simulink model "FSAC2021_V1"  (R2014a)
settings: Solver=FixedStepDiscrete  StartTime=0.0  StopTime=inf  FixedStep=0.0005  RelTol=1e-3
model workspace (MAT data in the model file):
  MCOS : class17 (value not decoded)
  MCOS : class17 (value not decoded)
  MCOS : class17 (value not decoded)
  MCOS : class17 (value not decoded)
  MCOS : class17 (value not decoded)
  MCOS : class17 (value not decoded)
  MCOS : class17 (value not decoded)
  MCOS : class17 (value not decoded)
  MCOS : class17 (value not decoded)
  MCOS : class17 (value not decoded)
  MCOS : class17 (value not decoded)
  MCOS : class17 (value not decoded)
  MCOS : class17 (value not decoded)
  MCOS : class17 (value not decoded)
  MCOS : class17 (value not decoded)
  MCOS : class17 (value not decoded)
  MCOS : class17 (value not decoded)
  MCOS : class17 (value not decoded)
  MCOS : class17 (value not decoded)
  BUZZER_START = 1
  MCOS : class17 (value not decoded)
  MCOS : class17 (value not decoded)
  MCOS : class17 (value not decoded)
  MCOS : class17 (value not decoded)
  MCOS : class17 (value not decoded)
  MCOS : class17 (value not decoded)
  MCOS : class17 (value not decoded)
  MCOS : class17 (value not decoded)
  MCOS : class17 (value not decoded)
  MCOS : class17 (value not decoded)
  MCOS : class17 (value not decoded)
  MCOS : class17 (value not decoded)
  MCOS : class17 (value not decoded)
  MCOS : class17 (value not decoded)
  MCOS : class17 (value not decoded)
  MCOS : class17 (value not decoded)
  MCOS : class17 (value not decoded)
  MCOS : class17 (value not decoded)
  MCOS : class17 (value not decoded)
  MCOS : class17 (value not decoded)
  MCOS : class17 (value not decoded)
  MCOS : class17 (value not decoded)
  MCOS : class17 (value not decoded)
  MCOS : class17 (value not decoded)
  MCOS : class17 (value not decoded)
  MCOS : class17 (value not decoded)
  MCOS : class17 (value not decoded)
  MCOS : class17 (value not decoded)
  MCOS : class17 (value not decoded)
  MCOS : class17 (value not decoded)
  MCOS : class17 (value not decoded)
  MCOS : class17 (value not decoded)
  MCOS : class17 (value not decoded)
  MCOS : class17 (value not decoded)
  MCOS : class17 (value not decoded)
  MCOS : class17 (value not decoded)
  MCOS : class17 (value not decoded)
  MCOS : class17 (value not decoded)
  Brake = 11
  MCOS : class17 (value not decoded)
  MCOS : class17 (value not decoded)
  MCOS : class17 (value not decoded)
  MCOS : class17 (value not decoded)
  MCOS : class17 (value not decoded)
  MCOS : class17 (value not decoded)
  MCOS : class17 (value not decoded)
  MCOS : class17 (value not decoded)
  Sensor_Acc_b = 101.85
  Sensor_Acc_k = -0.0185
  Str_Sen_Orig_Angle = -341
  MCOS : class17 (value not decoded)
  Tire_D = 0.47
  T = 0.05
libraries: simulink x189, ec55xxlib x135
(part 9 of 9)

== system FSAC2021_V1/VCU_CAN_Read/PCANB(BMS、DRIVE_MOTOR)/Str_Emergency /MOTEC_EMERGENCY/Str_PwrMod_TempHigh_Warning_Sub ==
  In1 : Inport
  Out1 : Outport
  wires:
  In1/1 -> Out1/1

== system FSAC2021_V1/VCU_CAN_Read/PCANB(BMS、DRIVE_MOTOR)/Str_Emergency /MOTEC_EMERGENCY/Str_Spd_Over_Alam_Sub ==
  In1 : Inport
  Out1 : Outport
  wires:
  In1/1 -> Out1/1

== system FSAC2021_V1/VCU_CAN_Read/PCANB(BMS、DRIVE_MOTOR)/Str_Emergency /MOTEC_EMERGENCY/Str_System_Error_Sub ==
  In1 : Inport
  Out1 : Outport
  wires:
  In1/1 -> Out1/1

== system FSAC2021_V1/VCU_CAN_Read/PCANB(BMS、DRIVE_MOTOR)/Str_Emergency /MOTEC_EMERGENCY/Str_UnderVolt_Warning_Sub ==
  In1 : Inport
  Out1 : Outport
  wires:
  In1/1 -> Out1/1

== system FSAC2021_V1/VCU_CAN_Read/Subsystem/BMS_HCU_INFO /BMS_HCU_INFO/BatAlmLv_Sub ==
  In1 : Inport
  Out1 : Outport
  wires:
  In1/1 -> Out1/1

== system FSAC2021_V1/VCU_CAN_Read/Subsystem/BMS_HCU_INFO /BMS_HCU_INFO/BatCurrent_Sub ==
  In1 : Inport
  Out1 : Outport
  wires:
  In1/1 -> Out1/1

== system FSAC2021_V1/VCU_CAN_Read/Subsystem/BMS_HCU_INFO /BMS_HCU_INFO/BatLife_Sub ==
  In1 : Inport
  Out1 : Outport
  wires:
  In1/1 -> Out1/1

== system FSAC2021_V1/VCU_CAN_Read/Subsystem/BMS_HCU_INFO /BMS_HCU_INFO/BatSoc_Sub ==
  In1 : Inport
  Out1 : Outport
  wires:
  In1/1 -> Out1/1

== system FSAC2021_V1/VCU_CAN_Read/Subsystem/BMS_HCU_INFO /BMS_HCU_INFO/BatSoh_Sub ==
  In1 : Inport
  Out1 : Outport
  wires:
  In1/1 -> Out1/1

== system FSAC2021_V1/VCU_CAN_Read/Subsystem/BMS_HCU_INFO /BMS_HCU_INFO/BatState_Sub ==
  In1 : Inport
  Out1 : Outport
  wires:
  In1/1 -> Out1/1

== system FSAC2021_V1/VCU_CAN_Read/Subsystem/BMS_HCU_INFO /BMS_HCU_INFO/BatVoltage_Sub ==
  In1 : Inport
  Out1 : Outport
  wires:
  In1/1 -> Out1/1

== system FSAC2021_V1/VCU_CAN_Read/Subsystem1/HEARTBEAT /MOTEC_HEARTBEAT/Heartbeat_info_Sub ==
  In1 : Inport
  Out1 : Outport
  wires:
  In1/1 -> Out1/1

== system FSAC2021_V1/VCU_CAN_Read/Subsystem2/MOTEC_STATUS /MOTEC_STATUS/Fault_Sub ==
  In1 : Inport
  Out1 : Outport
  wires:
  In1/1 -> Out1/1

== system FSAC2021_V1/VCU_CAN_Read/Subsystem2/MOTEC_STATUS /MOTEC_STATUS/Operation_Enabled_Sub ==
  In1 : Inport
  Out1 : Outport
  wires:
  In1/1 -> Out1/1

== system FSAC2021_V1/VCU_CAN_Read/Subsystem2/MOTEC_STATUS /MOTEC_STATUS/Quick_Stop_Sub ==
  In1 : Inport
  Out1 : Outport
  wires:
  In1/1 -> Out1/1

== system FSAC2021_V1/VCU_CAN_Read/Subsystem2/MOTEC_STATUS /MOTEC_STATUS/Ready_Switch_On_Sub ==
  In1 : Inport
  Out1 : Outport
  wires:
  In1/1 -> Out1/1

== system FSAC2021_V1/VCU_CAN_Read/Subsystem2/MOTEC_STATUS /MOTEC_STATUS/Switch_On_Disabled_Sub ==
  In1 : Inport
  Out1 : Outport
  wires:
  In1/1 -> Out1/1

== system FSAC2021_V1/VCU_CAN_Read/Subsystem2/MOTEC_STATUS /MOTEC_STATUS/Swtiched_On_Sub ==
  In1 : Inport
  Out1 : Outport
  wires:
  In1/1 -> Out1/1

== system FSAC2021_V1/VCU_CAN_Read/Subsystem2/MOTEC_STATUS /MOTEC_STATUS/Target_Reached_Sub ==
  In1 : Inport
  Out1 : Outport
  wires:
  In1/1 -> Out1/1

== system FSAC2021_V1/VCU_CAN_Read/Subsystem2/MOTEC_STATUS /MOTEC_STATUS/Voltage_Enabled_Sub ==
  In1 : Inport
  Out1 : Outport
  wires:
  In1/1 -> Out1/1

== system FSAC2021_V1/VCU_CAN_Read/Subsystem2/MOTEC_STATUS /MOTEC_STATUS/Warning_Sub ==
  In1 : Inport
  Out1 : Outport
  wires:
  In1/1 -> Out1/1

== stateflow chart FSAC2021_V1/DIAG/DIAG/Res_Diag/Subsystem/Chart1 ==
  state Normal
    en:
    Output = uint8(0);
  state Off
  state ON
  state On
    en:
    Output = uint8(1);
  (default) -> Normal
  Normal -> ON : [Input == 1]
  ON -> Off [order 1] : [Input == uint8(0)]
  Off -> ON : [Input == uint8(1)]
  ON -> On [order 2] : after(2,sec)
  data: Input input; Output output

== stateflow chart FSAC2021_V1/Controller/50ms_Duty/Visuality Check/Chart ==
  state Visuality_On
    en:Visual_Lights =uint8(1);
    Visual_Flag = uint8(1);
  state Visuality_Off
    en:Visual_Lights =uint8(0);
    Visual_Flag = uint8(0);
  (default) -> Visuality_On
  Visuality_On -> Visuality_Off : [after(2,sec)]
  data: Visual_Lights output uint8 size=3; Visual_Flag output uint8

== stateflow chart FSAC2021_V1/Controller/50ms_Duty/AS_Machine ==
  state Manual_Driving
    en:
    R2D = ON;
    Buzzer = BUZZER_START;
    ASSI_State = MANUAL_DRIVING;
  state AS_Off
    en:ASSI_State =AS_OFF;
    //System_48V_Relay = DISABLE;
    Blue_Light = OFF;
    Yellow_Light = OFF;
    //VCU_Valve = ON;
    du:Manual_R2D_Detect;
    Visuality_Check;
  state AS_Ready
    state Init
      en:
      ASSI_State = AS_READY;
      //System_48V_Relay = ENABLE;
    state Origin
      en:
      Yellow_Light = ON;
      Blue_Light = OFF;
    (default) -> Init
    Init -> Origin : [Origin_Flag == 1]
  state AS_Driving
    en:R2D = ON;
    ASSI_State = AS_DRIVING;
    Yellow_Light = BLINK;
    Blue_Light = OFF;
    Buzzer = BUZZER_START;
  state AS_Finished
    en:
    ASSI_State =AS_FINISH;
    R2D = OFF;
    Safety_Circuit_Relay = ON;
    //System_48V_Relay = OFF;
    Blue_Light = ON;
    Yellow_Light = OFF;
  state AS_Emergency
    en:
    ASSI_State = AS_EMERGENCY;
    R2D = OFF;
    Yellow_Light = OFF;
    Blue_Light = BLINK;
    Buzzer = BUZZER_EBS;
  (default) -> AS_Off
  AS_Off -> AS_Ready [order 2] : [LVMS&&ASMS && TS_Flag &&AMI_State != 0 &&...
      | AMI_State != MANUAL_MODE&&...
      | EBS_Flag==EBS_ARMED]
  AS_Ready -> AS_Off : [!ASMS ]
  Origin -> AS_Driving [order 1] : [after(5,sec) && Res_GO]
  AS_Off -> Manual_Driving [order 1] : [AMI_State == MANUAL_MODE&&...
      | TS_Flag&&...
      | !ASMS&&START_Flag&&Brake_Trigeer]
  Origin -> AS_Emergency [order 2] : [EBS_Flag==EBS_ENABLE]
  AS_Driving -> (junction 69) [order 2] : [EBS_Flag==EBS_ENABLE]
  (junction 69) -> AS_Emergency
  AS_Driving -> AS_Finished [order 1] : [Veh_Spd <= 1 &&...
      | Misson_Finished ]
  Manual_Driving -> AS_Off : [ !TS_Flag]
  AS_Finished -> AS_Emergency [order 1] : [ Res_EBS]
  AS_Emergency -> AS_Off : [!ASMS &&Buzzer_Overflag&&...
      |  EBS_Flag ==EBS_DISABLE]
  (junction 65) -> AS_Off
  AS_Finished -> (junction 64) [order 2]
  (junction 64) -> (junction 65) : [!ASMS  ]
  data: Blue_Light output uint8; Yellow_Light output uint8; Buzzer output uint8; TS_Flag input uint8; EBS_Flag input uint8; Safety_Circuit_Relay output uint8; ASSI_State output uint8; Veh_Spd input single; ASMS input uint8; ON parameter uint8; OFF parameter uint8; ENABLE parameter uint8; DISABLE parameter uint8; AS_OFF parameter uint8; AS_READY parameter uint8; AS_DRIVING parameter uint8; AS_FINISH parameter uint8; AS_EMERGENCY parameter uint8; BLINK parameter uint8; EBS_DISABLE parameter uint8; EBS_ARMED parameter uint8; EBS_ENABLE parameter uint8; R2D output uint8; MANUAL_DRIVING parameter uint8; MANUAL_MODE parameter uint8; LVMS input uint8; AMI_State input uint8; Res_EBS input uint8; Res_GO input uint8; START_Flag input uint8; Misson_Finished input uint8; Buzzer_Overflag input uint8; BUZZER_START parameter uint8; BUZZER_EBS parameter uint8; TRACKDRIVE parameter uint8; Brake_Trigeer input; Origin_Flag input
  events: Manual_R2D_Detect output FUNCTION_CALL_EVENT; Visuality_Check output FUNCTION_CALL_EVENT

== stateflow chart FSAC2021_V1/DIAG/DIAG/CAN_NODE_LOSTCOM/B_M_S_Check/Chart ==
  state Normal
    en:
    Output = uint8(1);
  state Off
  state ON
  state On
    en:
    Output = uint8(0);
  (default) -> Normal
  Normal -> ON : [Input == 0&&after(500,msec)]
  ON -> Off [order 1] : [Input == uint8(1)]
  Off -> ON : [Input == uint8(0)]
  ON -> On [order 2] : after(2,sec)
  data: Input input; Output output

== stateflow chart FSAC2021_V1/Controller/50ms_Duty/Subsystem/Chart ==
  state Task
    du:
    MODE = 3;%%车检任务
  state init
  state Manul
    du:
    MODE = 6;%手动模式
  state Driverless
    du:
    MODE = 2;%%无人驾驶模式
  (junction 15) -> Task
  init -> (junction 15) [order 3] : [AMI_Duty == 4 ]
  (default) -> init
  init -> Manul [order 1] : [AMI_Duty == 6]
  init -> Driverless [order 2] : [AMI_Duty == 1 || AMI_Duty == 2 || AMI_Duty == 3 || AMI_Duty == 5]
  data: AMI_Duty input; MODE output

== stateflow chart FSAC2021_V1/DIAG/DIAG/CAN_NODE_LOSTCOM/B_M_S_Check/Chart1 ==
  state Normal
    en:
    Output = uint8(1);
  state Off
  state ON
  state On
    en:
    Output = uint8(0);
  (default) -> Normal
  Normal -> ON : [Input == 0]
  ON -> Off [order 1] : [Input == uint8(1)]
  Off -> ON : [Input == uint8(0)]
  ON -> On [order 2] : after(2,sec)
  data: Input input; Output output

== stateflow chart FSAC2021_V1/Controller/200ms_Duty/Light_Subsystem2/Start_Horn/Chart ==
  state Start_Horn_ON
    en: Buzzer_Pin = ON;
  state Start_Horn_OFF
    en: Buzzer_Pin = OFF;
  (default) -> Start_Horn_ON
  Start_Horn_ON -> Start_Horn_OFF : [after(2,sec)]
  data: Buzzer_Pin output uint8; OFF parameter; ON parameter

== stateflow chart FSAC2021_V1/Controller/200ms_Duty/Light_Subsystem2/EBS_Horn/Chart ==
  state Horn
    state EBS_Horn_ON
      en: Buzzer_Pin = ON;
    state EBS_Horn_ON1
      en:Buzzer_Pin = OFF;
    (default) -> EBS_Horn_ON
    EBS_Horn_ON1 -> EBS_Horn_ON : [after(100,msec)]
    EBS_Horn_ON -> EBS_Horn_ON1 : [after(100,msec)]
  state EBS_Horn_OFF
    en: Buzzer_Pin = OFF;
    Buzzer_Overflag = ENABLE
  (default) -> Horn
  Horn -> EBS_Horn_OFF : [after(9,sec)]
  data: Buzzer_Pin output uint8; OFF parameter; ON parameter; Buzzer_Overflag output uint8; ENABLE parameter

== stateflow chart FSAC2021_V1/Controller/50ms_Duty/Subsystem/Subsystem2/Chart ==
  state init
    en:
    SteerCmd = 0;
    ACC = 200;
  state IN
    en:
    state Second
      du:
      SteerCmd = SteerCmd - 4.5;
    state Move
      du:
      SteerCmd = SteerCmd + 4.5;
    Move -> Second : [SteerCmd>=110]
    (default) -> Move
    Second -> Move : [SteerCmd <= -110]
  state end
    en:
    ACC = 0;
    SteerCmd = 0;
    Mission_Flag = uint8(1);
  (default) -> init
  init -> IN
  IN -> end : [after(27,sec)]
  data: Mission_Flag output; SteerCmd output; ACC output

== stateflow chart FSAC2021_V1/DIAG/DIAG/CAN_NODE_LOSTCOM/Subsystem1/Chart2 ==
  state Normal
    en:
    Output = uint8(1);
  state Off
  state ON
  state On
    en:
    Output = uint8(0);
  (default) -> Normal
  Normal -> ON : [Input == 0]
  ON -> Off [order 1] : [Input == uint8(1)]
  Off -> ON : [Input == uint8(0)]
  ON -> On [order 2] : after(2,sec)
  data: Input input; Output output

== stateflow chart FSAC2021_V1/DIAG/DIAG/CAN_NODE_LOSTCOM/Subsystem/Chart4 ==
  state Normal
    en:
    Output = uint8(1);
  state Off
  state ON
  state On
    en:
    Output = uint8(0);
  (default) -> Normal
  Normal -> ON : [Input == 0]
  ON -> Off [order 1] : [Input == uint8(1)]
  Off -> ON : [Input == uint8(0)]
  ON -> On [order 2] : after(2,sec)
  data: Input input; Output output

== matlab function FSAC2021_V1/DIAG/DIAG/EBS_Diag/MATLAB Function ==
  data: Assi_State input; ebs_failure output; ebs_gas1 input; ebs_gas2 input
function ebs_failure = fcn(Assi_State,ebs_gas1,ebs_gas2)
%#codegen
ebs_failure = 0;
if Assi_State == 2 || Assi_State == 3 
    if ebs_gas1 < 1000 
        ebs_failure = 1;
    elseif ebs_gas1 > 1000 && ebs_gas2 > 1000
        ebs_failure = 1;
    end
end
end

== matlab function FSAC2021_V1/Controller/50ms_Duty/EBS_Judge/MATLAB Function ==
  data: gas1 input; status output; gas2 input
function status = fcn(gas1,gas2)
%#codegen
status = 0;
if gas1== 1 ;
    status = 0;%%%disable
elseif gas1 == 0 && gas2 == 1;
    status = 1;%%%armed
elseif gas1 == 0  && gas2 == 0;
    status = 2;%%%enable
end

== stateflow chart FSAC2021_V1/Controller/SteerCtr/Chart ==
  state Pre_Operation_Mode
    en:
    NMT_nodeorder = uint8(1); //开启远程节点。
    NMT_nodectrl = uint8(0);//连接所有节点。
    du:TmtNMTCAN;
  state Init
  state Move
    state Goto
      du:TmtRPDO1CAN;
      Fault_Resrt = uint8(0);
      Enable_Operation_Ctrl = uint8(1);//允许操作。
      state Origin_Pos_Set
        en:
        Position_set = (Origin_Back_Angle);//电机回位角度赋值。
        New_Set_Point_Ctrl = uint8(0);
      state Origin_Aciton_Move
        en:
        New_Set_Point_Ctrl = uint8(1);//设置新位置点。
        Abs_or_Rel_Ctrl = uint8(0);//相对位置移动。
      (default) -> Origin_Pos_Set
      Origin_Aciton_Move -> Origin_Pos_Set [order 2]
      Origin_Pos_Set -> Origin_Aciton_Move
    state Motor_Enable
      du:TmtRPDO1CAN;
      state First
        en:
        Switch_On_Ctrl = uint8(0); //
        Enable_Voltage_Ctrl = uint8(1);//允许通电。
        Quick_Stop_Ctrl = uint8(1);//禁用快速停止。
      state Second
        en:Switch_On_Ctrl = uint8(1);// 伺服使能
      (default) -> First
      First -> Second
    state Motor_Move
      du:TmtRPDO1CAN;
      enflag = uint8(1);
      state Move_Position_Set
        en:
        Enable_Operation_Ctrl = uint8(1);//允许操作。
        Position_set = int16(Steer_Go_Angle);//期望电机角度赋值
        New_Set_Point_Ctrl = uint8(0);
        Abs_or_Rel_Ctrl = uint8(0);//相对位置移动。
      state Aciton_Move
        en:
        New_Set_Point_Ctrl = uint8(1);//设置新位置点。
        Abs_or_Rel_Ctrl = uint8(1);//绝对位置移动。
      (default) -> Move_Position_Set
      Move_Position_Set -> Aciton_Move
      Aciton_Move -> Move_Position_Set
    state Wait
    state Motor_Stanby
      du:TmtSDOCAN;
      Original_Flag = uint8(1);
      state Encoder1
        du:
        Encoder_Msg_Data[0] = 0x2B;
        Encoder_Msg_Data[1] = 0x04;//2004对象字典
        Encoder_Msg_Data[2] = 0x20;
        Encoder_Msg_Data[3] = 0x00;
        Encoder_Msg_Data[4] = 0x01;//编码器清零标志位为1
        Encoder_Msg_Data[5] = 0x00;
        exit:Encoder_Msg_Data[4] = 0x00;//编码器清零标志位为0
      (default) -> Encoder1
    (default) -> Motor_Enable
    Second -> Goto
    Origin_Aciton_Move -> Wait [order 1] : [abs(Origin_Back_Angle)<=2]
    Wait -> Origin_Aciton_Move [order 1] : [abs(Origin_Back_Angle) > 2]
    Wait -> Motor_Stanby [order 2] : [after(0.5,sec)]
    Encoder1 -> Motor_Move : [ASSI_State==uint8(3)]
  (default) -> Init
  Init -> Pre_Operation_Mode
  Pre_Operation_Mode -> Move : [Str_Status]
  data: NMT_nodeorder output uint8; NMT_nodectrl output uint8; Enable_Operation_Ctrl output uint8; Quick_Stop_Ctrl output uint8; Enable_Voltage_Ctrl output uint8; Halt_Ctrl output uint8; Switch_On_Ctrl output uint8; Abs_or_Rel_Ctrl output uint8; New_Set_Point_Ctrl output uint8; Position_set output single; Encoder_Msg_Data output uint8 size=6; Original_Flag output double; Origin_Back_Angle input single; Steer_Go_Angle input int8; ASSI_State input uint8; Str_Status input uint8; Fault_Resrt output double; flag output double; enflag output double
  events: TmtNMTCAN output FUNCTION_CALL_EVENT; TmtRPDO1CAN output FUNCTION_CALL_EVENT; TmtSDOCAN output FUNCTION_CALL_EVENT

== stateflow chart FSAC2021_V1/DIAG/DIAG/Analog_Sensor_Diag/Chart2 ==
  state Normal
    en:
    Output = uint8(0);
  state Off
  state ON
  state On
    en:
    Output = uint8(1);
  (default) -> Normal
  Normal -> ON : [Input == 1]
  ON -> Off [order 1] : [Input == uint8(0)]
  Off -> ON : [Input == uint8(1)]
  ON -> On [order 2] : after(0.5,sec)
  data: Input input; Output output

== stateflow chart FSAC2021_V1/DIAG/DIAG/Analog_Sensor_Diag/Chart3 ==
  state Normal
    en:
    Output = uint8(0);
  state Off
  state ON
  state On
    en:
    Output = uint8(1);
  (default) -> Normal
  Normal -> ON : [Input == 1]
  ON -> Off [order 1] : [Input == uint8(0)]
  Off -> ON : [Input == uint8(1)]
  ON -> On [order 2] : after(0.5,sec)
  data: Input input; Output output

== stateflow chart FSAC2021_V1/DIAG/DIAG/Analog_Sensor_Diag/Chart4 ==
  state Normal
    en:
    Output = uint8(0);
  state Off
  state ON
  state On
    en:
    Output = uint8(1);
  (default) -> Normal
  Normal -> ON : [Input == 1]
  ON -> Off [order 1] : [Input == uint8(0)]
  Off -> ON : [Input == uint8(1)]
  ON -> On [order 2] : after(0.5,sec)
  data: Input input; Output output

== stateflow chart FSAC2021_V1/DIAG/DIAG/Analog_Sensor_Diag/Chart1 ==
  state Normal
    en:
    Output = uint8(0);
  state Off
  state ON
  state On
    en:
    Output = uint8(1);
  (default) -> Normal
  Normal -> ON : [Input == 1]
  ON -> Off [order 1] : [Input == uint8(0)]
  Off -> ON : [Input == uint8(1)]
  ON -> On [order 2] : after(0.5,sec)
  data: Input input; Output output

== stateflow chart FSAC2021_V1/DIAG/DIAG/Analog_Sensor_Diag/Chart5 ==
  state Normal
    en:
    Output = uint8(0);
  state Off
  state ON
  state On
    en:
    Output = uint8(1);
  (default) -> Normal
  Normal -> ON : [Input == 1]
  ON -> Off [order 1] : [Input == uint8(0)]
  Off -> ON : [Input == uint8(1)]
  ON -> On [order 2] : after(0.5,sec)
  data: Input input; Output output

== stateflow chart FSAC2021_V1/DIAG/DIAG/CAN_NODE_LOSTCOM/Subsystem1/Chart3 ==
  state Normal
    en:
    Output = uint8(1);
  state Off
  state ON
  state On
    en:
    Output = uint8(0);
  (default) -> Normal
  Normal -> ON : [Input == 0]
  ON -> Off [order 1] : [Input == uint8(1)]
  Off -> ON : [Input == uint8(0)]
  ON -> On [order 2] : after(2,sec)
  data: Input input; Output output

== stateflow chart FSAC2021_V1/DIAG/DIAG/CAN_NODE_LOSTCOM/Subsystem1/Chart4 ==
  state Normal
    en:
    Output = uint8(1);
  state Off
  state ON
  state On
    en:
    Output = uint8(0);
  (default) -> Normal
  Normal -> ON : [Input == 0]
  ON -> Off [order 1] : [Input == uint8(1)]
  Off -> ON : [Input == uint8(0)]
  ON -> On [order 2] : after(2,sec)
  data: Input input; Output output

== stateflow chart FSAC2021_V1/Controller/BCU_Controller/BCU_Strategy ==
  state RunMode
    state Init
      en:Brk_Mtr_Enable; ///制动电机使能
    state Tozeros
      en:
      Brk_Ctrl_State=uint8(2);//制动回位
    state Move
      en:Allow_Ctrl_Flg=ENABLE;
      Brk_Ctrl_State = BRK_MOVE;
    state BackOrigin
      en:Brk_Mtr_BackOrigin;///转向电机回位
      Brk_Ctrl_State=uint8(1);//制动占用
    (default) -> Init
    Init -> BackOrigin : [Brk_Mtr_Enable_Flg && ASSI_State == 2]
    BackOrigin -> Tozeros : [ASSI_State==3]
    Tozeros -> Move : after(0.5,sec)
  state Idle
  (default) -> Idle
  Idle -> RunMode
  data: Brk_Mtr_Enable_Flg input uint8; BRK_DISPSENS_LOWLIMIT parameter single; Allow_Ctrl_Flg output uint8 =0; ENABLE parameter uint8; Brk_Ctrl_State output uint8; BRK_ENGAGED parameter uint8; BRK_TOZERO parameter uint8; BRK_MOVE parameter uint8; DISABLE parameter uint8; ASSI_State input; Brk_Mtr_Origin_Flag input
  events: Brk_Mtr_BackOrigin output FUNCTION_CALL_EVENT; Brk_Mtr_Enable output FUNCTION_CALL_EVENT

== stateflow chart FSAC2021_V1/DIAG/DIAG/ACC/Enabled Subsystem/Chart ==
  state Action
    en:
    Acc_Flag = 1;
  state Init
    en:
    Acc_Flag = 0;
  state Action1
    en:
    Acc_Flag = 0;
  (default) -> Init
  Init -> Action : [liquid_presuress > 200 && Acc >= 25 && after(500,msec)]
  Action1 -> Action : [liquid_presuress > 200 && Acc >= 25 && after(500,msec)]
  Action -> Action1 : [Acc <= 5]
  data: liquid_presuress input; Acc input; Acc_Flag output

== matlab function FSAC2021_V1/Controller/50ms_Duty/Subsystem1/MATLAB Function ==
  data: LVMS input; Relay_48V output; ASMS input; ASSI_State input
function Relay_48V = fcn(LVMS,ASMS,ASSI_State)
%#codegen
Relay_48V = 0;
if LVMS == 1 && ASMS == 1
    Relay_48V = 1;
if LVMS == 0 || ASMS == 0 || ASSI_State == 0 || ASSI_State == 4
    Relay_48V = 0;
end

end
